simulink model "pam_generator"  (R2021a)
settings: Solver=VariableStepAuto  StartTime=0.0  StopTime=0.1  RelTol=1e-3
settings Model: Creator=Bremdow  LastModifiedBy=Bremdow

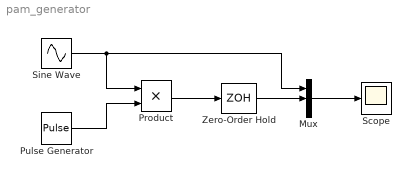
== system pam_generator ==
  Mux : Mux  Inputs=3
  Product : Product
  Pulse Generator : DiscretePulseGenerator  PulseType=Time based  Period=0.0001  PulseWidth=5
  Scope : Scope
  Sine Wave : Sin  Frequency=1000  SampleTime=0
  Zero-Order Hold : ZeroOrderHold  SampleTime=-1
  wires:
  Product/1 -> Zero-Order Hold/1
  Sine Wave/1 -> Mux/1, Product/1
  Pulse Generator/1 -> Product/2
  Mux/1 -> Scope/1
  Zero-Order Hold/1 -> Mux/2
